simulink model "MONZA_fuzzy_delia_3"  (R2025b)
settings: Solver=FixedStepDiscrete  StartTime=0  StopTime=20  FixedStep=0.033  RelTol=1e-3
InitFcn:
  | cargar_fis;
libraries: fuzblock x1
settings Model: Creator=christian  LastModifiedBy=delia
settings SolverCC: AlgebraicLoopSolver=TrustRegion
settings DataIOCC: ReturnWorkspaceOutputs=off
settings DebuggingCC: UnconnectedInputMsg=warning  UnconnectedOutputMsg=warning  UnconnectedLineMsg=warning  ArithmeticOperatorsInVariantConditions=warning
settings ModelReferenceCC: EnableRefExpFcnMdlSchedulingChecks=on
settings SFSimCC: SimUseLocalCustomCode=off  CustomCodeUndefinedFunction=UseInterfaceOnly
settings RTWCC: RTWUseLocalCustomCode=off  GPUComputeCapability=3.5

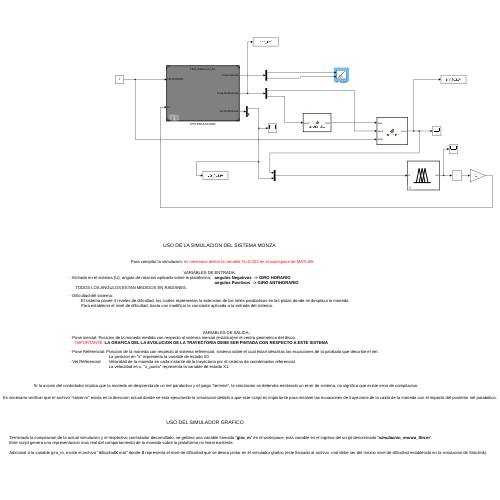
[thumbnail: Simulink's stored preview of the top-level diagram]
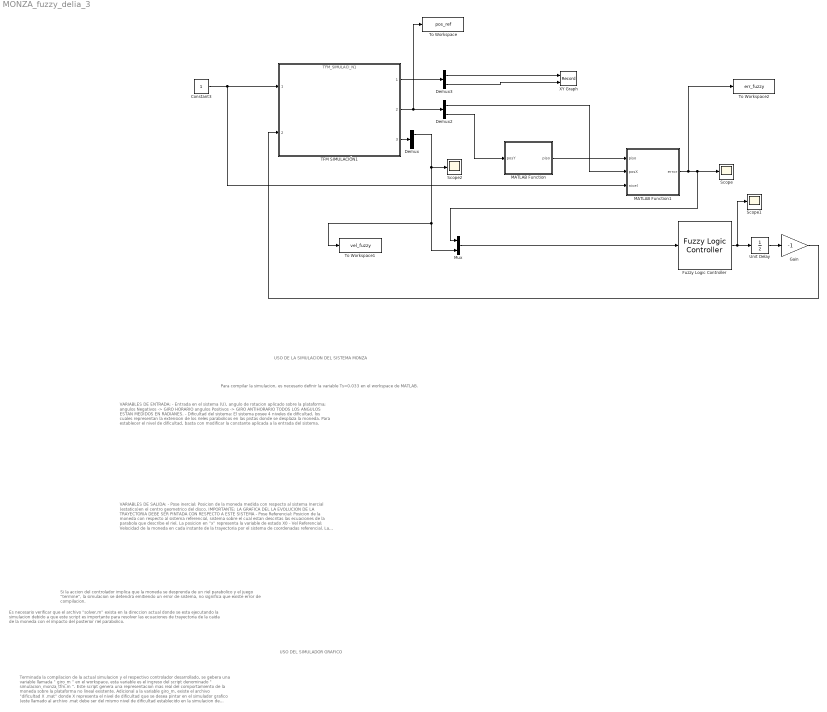
== system MONZA_fuzzy_delia_3 ==
  note: Es necesario verificar que el archivo "solver.m" exista en la direccion actual donde se esta ejecutando la simulacion debido a que este script es importante para resolver las ecuaciones de trayectoria de la caida de la moneda con el impacto del posterior riel parabolico.
  note: Si la accion del controlador implica que la moneda se desprenda de un riel parabolico y el juego "termine", la simulacion se detendra emitiendo un error de sistema, no significa que existe error de compilacion.
  note: Para compilar la simulacion, es necesario definir la variable Ts=0.033 en el workspace de MATLAB.
  note: VARIABLES DE ENTRADA:
      | - Entrada en el sistema (U), angulo de rotacion aplicado sobre la plataforma; angulos Negativos -> GIRO HORARIO
      | angulos Positivos -> GIRO ANTIHORARIO
      | TODOS LOS ANGULOS ESTAN MEDIDOS EN RADIANES.
      |
      | - Dificultad del sistema:
      | El sistema posee 4 niveles de dificultad, los cuales representan la extension de los rieles parabolicos en las pistas donde se desplaza la moneda.
      | Para establecer el nivel de dificultad, basta con modificar la constante aplicada a la entrada del sistema.
  note: USO DE LA SIMULACION DEL SISTEMA MONZA
  note: VARIABLES DE SALIDA:
      | - Pose inercial: Posicion de la moneda medida con respecto al sistema Inercial (estatico)en el centro geometrico del disco.
      | IMPORTANTE: LA GRAFICA DEL LA EVOLUCION DE LA TRAYECTORIA DEBE SER PINTADA CON RESPECTO A ESTE SISTEMA
      |
      | - Pose Referencial: Posicion de la moneda con respecto al sistema referencial, sistema sobre el cual estan descritas las ecuaciones de la parabola que describe el riel.
      | La posicion en "x" representa la variable de estado X0
      | - Vel Referencial: Velocidad de la moneda en cada instante de la trayectoria por el sistema de coordenadas referencial.
      | La velocidad en x, "x_punto" representa la variable de estado X1.
  note: USO DEL SIMULADOR GRAFICO
  note: Terminada la compilacion de la actual simulacion y el respectivo controlador desarrollado, se gebera una variable llamada " giro_m " en el workspace, esta variable es el ingreso del script denominado " simulacion_monza_tfm.m ".
      | Este script genera una representacion mas real del comportamiento de la moneda sobre la plataforma no lineal existente.
      |
      | Adicional a la variable giro_m, existe el archivo "dificultad X .mat" donde X representa el nivel de dificultad que se desea pintar en el simulador grafico (este llamado al archivo .mat debe ser del mismo nivel de dificultad establecido en la simulacion de Simulink)
  Constant3 : Constant
  Demux : Demux  Outputs=2
  Demux2 : Demux  Outputs=2
  Demux3 : Demux  Outputs=2
  Fuzzy Logic Controller : fuzblock/Fuzzy Logic  Controller  FIS=fisController  OutputSampleNumber=101  DataType=double  UseLookupTable=off  NumBreakpoints=10  FuzzifiedInputs=off  RuleFiringStrengths=off  RuleOutputs=off  AggregatedOutputs=off  SimulateUsing=Interpreted execution  OutOfRangeInputValueMessage=warning  NoRuleFiredMessage=warning  EmptyOutputFuzzySetMessage=warning
  Gain : Gain  Gain=-1
  MATLAB Function : MATLAB Function  TreatAsAtomicUnit=on
  MATLAB Function1 : MATLAB Function  TreatAsAtomicUnit=on
  Mux : Mux  Inputs=2
  Scope : Scope
      settings: ActiveDisplayYMinimum=-0.22893228225067025  ActiveDisplayYMaximum=0.16039054025603233
  Scope1 : Scope
      settings: ActiveDisplayYMinimum=-0.24600738770357777  ActiveDisplayYMaximum=0.24603736650805766
  Scope2 : Scope
      settings: ActiveDisplayYMinimum=-1  ActiveDisplayYMaximum=1  DataLoggingVariableName=ScopeData2
  TFM SIMULACIÓN1 : ModelReference  ModelNameDialog=TFM_SIMULACI_N1.slx  UsingDefaultArgumentValue=0,0  SimulationMode=Normal  ModelReferenceVersion=17.0  Gain=0.05  Gain2=0.0223
  To Workspace : ToWorkspace  VariableName=pos_ref  SaveFormat=Timeseries  SampleTime=-1
  To Workspace1 : ToWorkspace  VariableName=vel_fuzzy  SaveFormat=Timeseries  SampleTime=-1
  To Workspace2 : ToWorkspace  VariableName=err_fuzzy  SaveFormat=Timeseries  SampleTime=-1
  Unit Delay : UnitDelay  SampleTime=0.033  HasFrameUpgradeWarning=on
  XY Graph : Record  NumPorts=2.0  FileSettingsInternal="{\"entries\":[{\"content\":{\"excelSettings\":{\"content\":{},\"type\":\"Streamout.ExcelSettings\"},\"parquetSettings\":{\"content\":{},\"type\":\"Streamout.ParquetSettings\"}},\"type\":\"Streamout.FileSettingStorage\",\"uuid\":\"\"}],\"packageUris\":[\"http:\\/\\/schema.mathworks.com\\/mf0\\/streamout_blocks\\/R2020a\"],\"version\":\"1.0\"}"  FrameSettings=[0, 0]  Layout=[1 1]  SignalsInternal="{\"entries\":[{\"content\":{\"signals\":[{\"content\":{\"blockPath\":[],\"dimensions\":[1],\"domain\":\"\",\"lineColor\":\"#a2142f\",\"plots\":[ 1 ],\"port\":1,\"signalID\":1,\"signalName\":\"XY Graph:1\"},\"type\":\"RecordBlkView.Signal\",\"uuid\":\"\"},{\"content\":{\"blockPath\":[],\"dimensions\":[1],\"domain\":\"\",\"lineColor\":\"#139fff\",\"plots\":[ 1 ],\"port\":2,\"signalID\":2,\"signalName\":\"XY Graph:2\"},\"type\":\"RecordBlkView.Signal\",\"uuid\":\"\"}]},\"type\":\"RecordBlkView.InputSignals\",\"uuid\":\"\"}],\"packageUris\":[\"http:\\/\\/schema.mathworks.com\\/mf0\\/streamout_blocks\\/R2020a\"],\"version\":\"1.0\"}"  VisualizationBindings="{\"xyplotplugin\":{\"info\":[{\"series\":[{\"bindingParametersList\":[{\"parameter\":\"X-Axis\",\"signalID\":1,\"signalName\":\"XY Graph:1\"},{\"parameter\":\"Y-Axis\",\"signalID\":2,\"signalName\":\"XY Graph:2\"}],\"seriesID\":0}],\"subplotID\":1}]}}"  CompatibilityTag=XY
  wires:
  TFM SIMULACIÓN1/2 -> To Workspace/1, Demux2/1
  Constant3/1 -> MATLAB Function1/3(nivel), TFM SIMULACIÓN1/1
  Demux2/2 -> MATLAB Function/1(posY)
  MATLAB Function/1(piso) -> MATLAB Function1/1(piso)
  Demux2/1 -> MATLAB Function1/2(posX)
  MATLAB Function1/1(error) -> To Workspace2/1, Mux/1, Scope/1
  Mux/1 -> Fuzzy Logic Controller/1
  Fuzzy Logic Controller/1 -> Scope1/1, Unit Delay/1
  TFM SIMULACIÓN1/3 -> Demux/1
  Demux/1 -> Scope2/1, To Workspace1/1, Mux/2
  Unit Delay/1 -> Gain/1
  Gain/1 -> TFM SIMULACIÓN1/2
  TFM SIMULACIÓN1/1 -> Demux3/1
  Demux3/1 -> XY Graph/1
  Demux3/2 -> XY Graph/2

== matlab function MONZA_fuzzy_delia_3/MATLAB Function ==
  data: posY input; piso output
function piso = calcula_piso(posY)
%CALCULA_PISO  Devuelve el piso (1..7) según la altura Y referencial de la moneda.
%   Los 7 pisos son parábolas apiladas y = -0.54*x^2 + C, con las constantes C
%   (alturas de vértice) sacadas de make_ref_dif_aware.m:
%       h_values = [0.1143, 0.0686, 0.03, -0.03, -0.0686, -0.1143, -0.16];
%   Los umbrales son los puntos medios entre vértices consecutivos.
%   posY debe estar en el sistema REFERENCIAL (Pose Referencial de la planta).

    % Umbrales (puntos medios entre alturas de piso), de arriba (piso 1) a abajo.
    if     posY >=  0.09145    % por encima del punto medio piso 1/2
        piso = 1;
    elseif posY >=  0.04930
        piso = 2;
    elseif posY >=  0.00000
        piso = 3;
    elseif posY >= -0.04930
        piso = 4;
    elseif posY >= -0.09145
        piso = 5;
    elseif posY >= -0.13715
        piso = 6;
    else                       % por debajo del punto medio piso 6/7
        piso = 7;
    end
end

== matlab function MONZA_fuzzy_delia_3/MATLAB Function1 ==
  data: piso input; error output; posX input; nivel input
function error = controller(piso, posX, nivel)
      metas_x = [ ...
          0,        0,        0,        0,        0,        0,      -0.02554;  ... % dif 1
          0.06211, -0.04758,  0.04969, -0.04847,  0.04406, -0.05409,-0.02554;  ... % dif 2
          0.12394, -0.09503,  0.09924, -0.0968,   0.08803, -0.108,  -0.02554;  ... % dif 3
          0.12394, -0.14224,  0.14851, -0.14488,  0.1318,  -0.108,  -0.02554 ]; ... % dif 4
          
      % margen por dificultad (sentido de avance via signo).
      % dif1/2 POSITIVO = empujar más allá de la puerta (puertas centradas).
      % dif3/4 NEGATIVO = apuntar POR DENTRO de la puerta (puertas muy afuera; la
      % moneda llega con inercia de sobra, el empuje sólo causaba sobrepaso).
      margenes = [0.08, 0.03, -0.02, -0.07];
      signo    = [1, -1, 1, -1, 1, -1, -1];
      
      p = double(piso);
      if p < 1, p = 1; elseif p > 7, p = 7; end
      d = double(nivel);
      if d < 1, d = 1; elseif d > 4, d = 4; end
      p = round(p); d = round(d);
      
      margen = margenes(d);
      meta_x = metas_x(d, p) + margen * signo(p);
      error  = posX - meta_x;
  end
